simulink model "Project_HIL_Case_3"  (R2018b)
settings: Solver=ode5  StartTime=0.0  StopTime=180  FixedStep=0.01  RelTol=1e-3
InitFcn:
  | Initial_Data_Case_3
values from neighbouring files (symbols this model uses):
  alpha1 = 0.5    [Initial_Data_Case_3.m]
  alpha2 = 0.5    [Initial_Data_Case_3.m]
  alpha3 = 0.5    [Initial_Data_Case_3.m]
  gammadot_t = 0*pi/180    (= 0)    [Initial_Data_Case_3.m]
  landa1 = 1    [Initial_Data_Case_3.m]
  landa2 = 1    [Initial_Data_Case_3.m]
  landa3 = 1    [Initial_Data_Case_3.m]
  Vg_t = 10    [Initial_Data_Case_3.m]
undefined symbols (not defined in the file or in its folder): Serial_Port, Standard_Devices
libraries: svdutilitieslib x2, sldrtlib x2
settings Model: Creator=AmiR_KhaN  LastModifiedBy=AmiR_KhaN
settings DataIOCC: ReturnWorkspaceOutputs=on
settings RTWCC: Description=Simulink Desktop Real-Time  SystemTargetFile=sldrt.tlc  TemplateMakefile=sldrt.tmf  RTWCompilerOptimization=on
settings CodeAppCC: MaxIdLength=95
settings SimulinkDesktopRealTimeCC: TargetPreCompLibLocation=E:\programmes\newmatlab\toolbox\sldrt\lib\win64

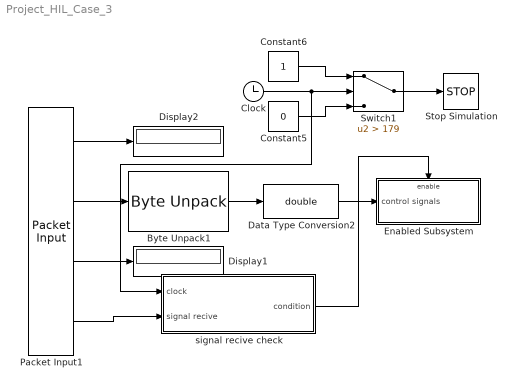
== system Project_HIL_Case_3 ==
  Byte Unpack1 : svdutilitieslib/Byte Unpack  dimensions={[3]}  datatypes={'single'}  byteAlign=1  blockPlatform=arduinoert
      settings: SourceProductBaseCode=ARDUINO,ML_ARDUINO,ECCORTEXA,ECCORTEXR,SC_BEAGLEBONE_BLUE,EC_FREEDOM_BOARD,EC_FRDM_K64F,INTEL_BLOCKSET,MICROBIT,NUCLEO,PX4AUTOPILOTS,RASPPIIO,STMICRODIS,TIC2000,XILINX_BLOCKSET
  Clock : Clock
  Constant5 : Constant  Value=0
  Constant6 : Constant
  Data Type Conversion2 : DataTypeConversion  OutDataTypeStr=double
  Display1 : Display
  Display2 : Display
  Enabled Subsystem : Subsystem  TreatAsAtomicUnit=on
  Packet Input1 : sldrtlib/Packet Input  SampleTime=0.01  MaxMissedTicks=10  ShowMissedTicks=off  YieldWhenWaiting=off  DrvName=Standard_Devices/Serial_Port  DrvAddress=5  DrvOptions=[9600 8 0 0 0 0 0 0]  PacketSize=14  DataTypes={'1*uint8','12*uint8','1*uint8'}  ShowReady=on  ShowError=off  PacketID=1  ByteOrder=1  ShowTimestamp=off
      settings: AttributesFormatString=Serial Port [5]
  Stop Simulation : Stop
  Switch1 : Switch  Criteria=u2 > Threshold  Threshold=179
  signal recive check : Subsystem
  wires:
  Packet Input1/1 -> Display2/1
  Packet Input1/3 -> Display1/1
  Clock/1 -> signal recive check/1(clock), Switch1/2
  Constant5/1 -> Switch1/3
  Data Type Conversion2/1 -> Enabled Subsystem/1(control signals)
  Constant6/1 -> Switch1/1
  Byte Unpack1/1 -> Data Type Conversion2/1
  Switch1/1 -> Stop Simulation/1
  Packet Input1/2 -> Byte Unpack1/1
  Packet Input1/4 -> signal recive check/2(signal recive)
  signal recive check/1(condition) -> Enabled Subsystem/Enable

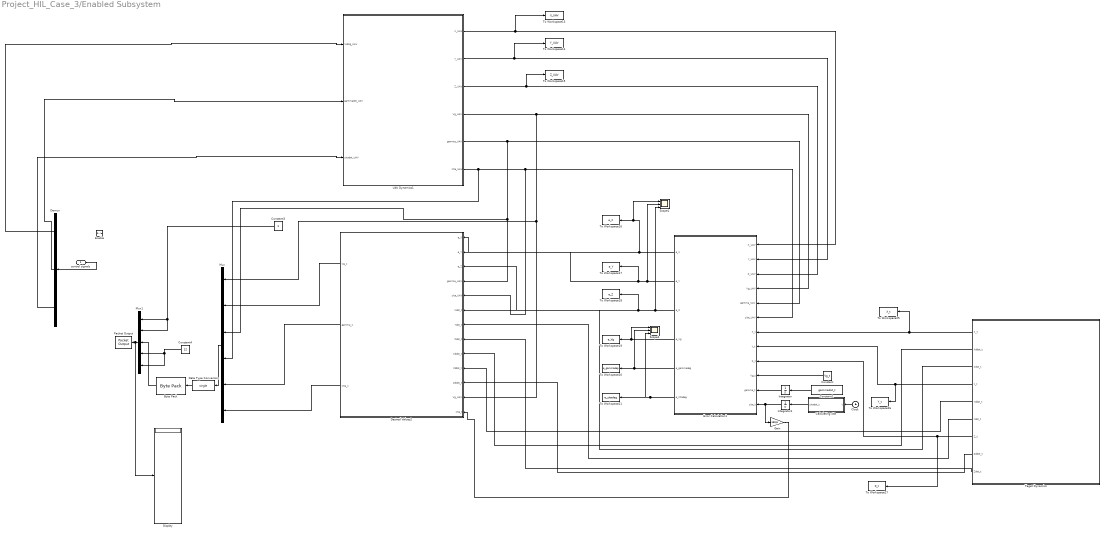
== system Project_HIL_Case_3/Enabled Subsystem ==
  control signals : Inport
  Enable : EnablePort
  Byte Pack : svdutilitieslib/Byte Pack  maskPackedDataType=uint8  datatypes={'single'}  byteAlign=4  blockPlatform=arduinoert
      settings: SourceProductBaseCode=ARDUINO,ML_ARDUINO,ECCORTEXA,ECCORTEXR,SC_BEAGLEBONE_BLUE,EC_FREEDOM_BOARD,EC_FRDM_K64F,INTEL_BLOCKSET,MICROBIT,NUCLEO,PX4AUTOPILOTS,RASPPIIO,STMICRODIS,TIC2000,XILINX_BLOCKSET
  Calculating zita : MATLAB Function  TreatAsAtomicUnit=on
  Clock : Clock
  Constant : Constant  Value=Vg_t
  Constant1 : Constant  Value=gammadot_t
  Constant3 : Constant  OutDataTypeStr=uint8
  Constant4 : Constant  Value=12  OutDataTypeStr=uint8
  Data Type Conversion : DataTypeConversion  OutDataTypeStr=single
  Demux : Demux  Outputs=3
  Desired Values2 : Subsystem
  Display : Display
  Error Calculation1 : MATLAB Function  TreatAsAtomicUnit=on
  Gain : Gain  Gain=180/pi
  Integrator : Integrator  InitialCondition=45*pi/180
  Integrator1 : Integrator  InitialCondition=0*pi/180
  Mux : Mux  Inputs=6
  Mux1 : Mux  Inputs=5
  Packet Output : sldrtlib/Packet Output  SampleTime=0.01  MaxMissedTicks=10  ShowMissedTicks=off  YieldWhenWaiting=off  DrvName=Standard_Devices/Serial_Port  DrvAddress=5  DrvOptions=[9600 8 0 0 0 0 0 0]  PacketSize=28  DataTypes='28*uint8'  ShowReady=off  ShowError=off  PacketID=1  ByteOrder=1  InitialValue=[]  FinalValue=[]
      settings: AttributesFormatString=Serial Port [5]
  Scope1 : Scope  NumInputPorts=3
  Scope2 : Scope  NumInputPorts=3
  Taget Dynamics : Subsystem
  To Workspace13 : ToWorkspace  VariableName=X_UAV  SaveFormat=Timeseries  SampleTime=-1
  To Workspace14 : ToWorkspace  VariableName=Y_UAV  SaveFormat=Timeseries  SampleTime=-1
  To Workspace15 : ToWorkspace  VariableName=Z_UAV  SaveFormat=Timeseries  SampleTime=-1
  To Workspace16 : ToWorkspace  VariableName=e_X  SaveFormat=Timeseries  SampleTime=-1
  To Workspace17 : ToWorkspace  VariableName=e_Y  SaveFormat=Timeseries  SampleTime=-1
  To Workspace18 : ToWorkspace  VariableName=e_Z  SaveFormat=Timeseries  SampleTime=-1
  To Workspace19 : ToWorkspace  VariableName=e_Vg  SaveFormat=Timeseries  SampleTime=-1
  To Workspace20 : ToWorkspace  VariableName=e_gammadeg  SaveFormat=Timeseries  SampleTime=-1
  To Workspace21 : ToWorkspace  VariableName=e_zitadeg  SaveFormat=Timeseries  SampleTime=-1
  To Workspace25 : ToWorkspace  VariableName=X_t  SaveFormat=Timeseries  SampleTime=-1
  To Workspace26 : ToWorkspace  VariableName=Y_t  SaveFormat=Timeseries  SampleTime=-1
  To Workspace27 : ToWorkspace  VariableName=Z_t  SaveFormat=Timeseries  SampleTime=-1
  UAV Dynamics1 : Subsystem
  wires:
  Desired Values2/3(zita_c) -> Mux/6
  control signals/1 -> Demux/1
  Constant4/1 -> Mux1/5, Mux1/4
  Demux/2 -> UAV Dynamics1/2(gammadot_UAV)
  Demux/1 -> UAV Dynamics1/1(Vdotg_UAV)
  Demux/3 -> UAV Dynamics1/3(zitadot_UAV)
  Data Type Conversion/1 -> Byte Pack/1
  Mux1/1 -> Display/1, Packet Output/1
  Mux/1 -> Data Type Conversion/1
  Byte Pack/1 -> Mux1/3
  Desired Values2/1(Vg_c) -> Mux/2
  Desired Values2/2(gamma_c) -> Mux/5
  UAV Dynamics1/6(zita_UAV) -> Mux/4, Desired Values2/5(zita_UAV), Error Calculation1/6(zita_UAV)
  Taget Dynamics/7(Z_t) -> To Workspace27/1, Error Calculation1/9(Z_t)
  Taget Dynamics/1(X_t) -> To Workspace25/1, Error Calculation1/7(X_t)
  Taget Dynamics/5(Yddot_t) -> Desired Values2/10(Yddot_t)
  Taget Dynamics/2(Xddot_t) -> Desired Values2/9(Xddot_t)
  Constant/1 -> Error Calculation1/10(Vg_t)
  Clock/1 -> Calculating zita/1(t)
  Taget Dynamics/6(Ydot_t) -> Desired Values2/7(Ydot_t)
  Taget Dynamics/4(Y_t) -> To Workspace26/1, Error Calculation1/8(Y_t)
  Taget Dynamics/9(Zdot_t) -> Desired Values2/8(Zdot_t)
  Taget Dynamics/3(Xdot_t) -> Desired Values2/6(Xdot_t)
  UAV Dynamics1/3(Z_UAV) -> To Workspace15/1, Error Calculation1/3(Z_UAV)
  Constant1/1 -> Integrator/1
  Taget Dynamics/8(Zddot_t) -> Desired Values2/11(Zddot_t)
  Calculating zita/1(zitadot_t) -> Integrator1/1
  UAV Dynamics1/2(Y_UAV) -> To Workspace14/1, Error Calculation1/2(Y_UAV)
  Gain/1 -> Desired Values2/13(zita_t)
  UAV Dynamics1/1(X_UAV) -> To Workspace13/1, Error Calculation1/1(X_UAV)
  Integrator1/1 -> Error Calculation1/12(zita_t), Gain/1
  UAV Dynamics1/5(gamma_UAV) -> Mux/3, Desired Values2/4(gamma_UAV), Error Calculation1/5(gamma_UAV)
  Integrator/1 -> Error Calculation1/11(gamma_t)
  UAV Dynamics1/4(Vg_UAV) -> Mux/1, Desired Values2/12(Vg_UAV), Error Calculation1/4(Vg_UAV)
  Constant3/1 -> Mux1/2, Mux1/1
  Error Calculation1/4(e_Vg) -> Scope2/1, To Workspace19/1
  Error Calculation1/6(e_zitadeg) -> Scope2/3, To Workspace21/1
  Error Calculation1/5(e_gammadeg) -> Scope2/2, To Workspace20/1
  Error Calculation1/1(e_X) -> Desired Values2/1(e_X), Scope1/1, To Workspace16/1
  Error Calculation1/3(e_Z) -> Scope1/3, Desired Values2/3(e_Z), To Workspace18/1
  Error Calculation1/2(e_Y) -> Scope1/2, Desired Values2/2(e_Y), To Workspace17/1

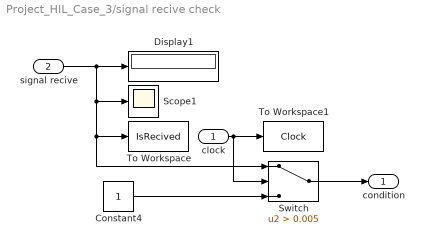
== system Project_HIL_Case_3/signal recive check ==
  clock : Inport
  signal recive : Inport  Port=2
  Constant4 : Constant
  Display1 : Display
  Scope1 : Scope
  Switch : Switch  Criteria=u2 > Threshold  Threshold=0.005
  To Workspace : ToWorkspace  VariableName=IsRecived  SampleTime=-1
  To Workspace1 : ToWorkspace  VariableName=Clock  SampleTime=-1
  condition : Outport
  wires:
  signal recive/1 -> Switch/1, To Workspace/1, Scope1/1, Display1/1
  Switch/1 -> condition/1
  clock/1 -> Switch/2, To Workspace1/1
  Constant4/1 -> Switch/3

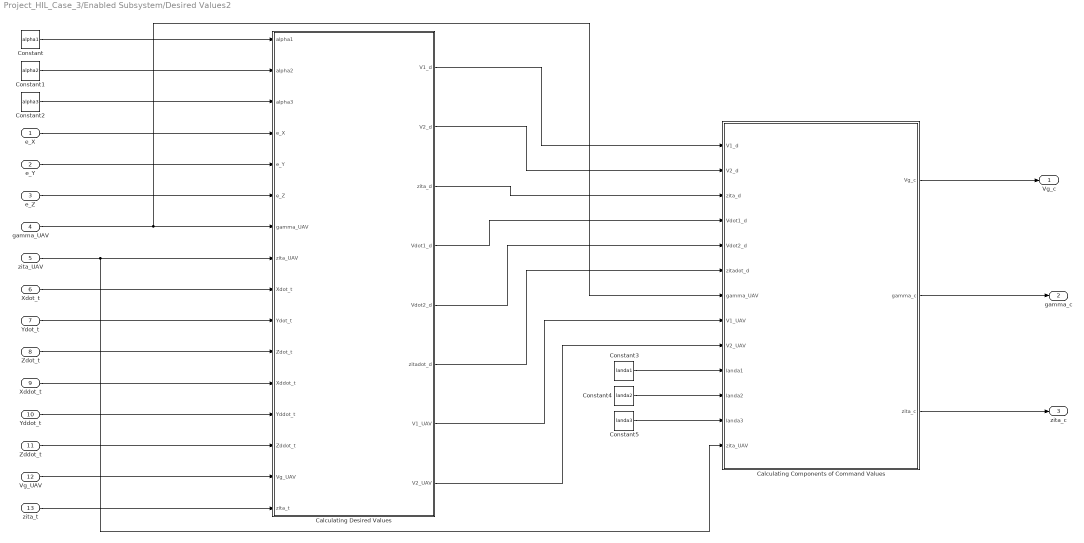
== system Project_HIL_Case_3/Enabled Subsystem/Desired Values2 ==
  e_X : Inport
  e_Y : Inport  Port=2
  e_Z : Inport  Port=3
  gamma_UAV : Inport  Port=4
  zita_UAV : Inport  Port=5
  Xdot_t : Inport  Port=6
  Ydot_t : Inport  Port=7
  Zdot_t : Inport  Port=8
  Xddot_t : Inport  Port=9
  Yddot_t : Inport  Port=10
  Zddot_t : Inport  Port=11
  Vg_UAV : Inport  Port=12
  zita_t : Inport  Port=13
  Calculating Components of Command Values : MATLAB Function  TreatAsAtomicUnit=on
  Calculating Desired Values : MATLAB Function  TreatAsAtomicUnit=on
  Constant : Constant  Value=alpha1
  Constant1 : Constant  Value=alpha2
  Constant2 : Constant  Value=alpha3
  Constant3 : Constant  Value=landa1
  Constant4 : Constant  Value=landa2
  Constant5 : Constant  Value=landa3
  Vg_c : Outport  VectorParamsAs1DForOutWhenUnconnected=off
  gamma_c : Outport  Port=2  VectorParamsAs1DForOutWhenUnconnected=off
  zita_c : Outport  Port=3  VectorParamsAs1DForOutWhenUnconnected=off
  wires:
  Constant/1 -> Calculating Desired Values/1(alpha1)
  Constant1/1 -> Calculating Desired Values/2(alpha2)
  Constant2/1 -> Calculating Desired Values/3(alpha3)
  e_X/1 -> Calculating Desired Values/4(e_X)
  e_Y/1 -> Calculating Desired Values/5(e_Y)
  e_Z/1 -> Calculating Desired Values/6(e_Z)
  gamma_UAV/1 -> Calculating Desired Values/7(gamma_UAV), Calculating Components of Command Values/7(gamma_UAV)
  zita_UAV/1 -> Calculating Desired Values/8(zita_UAV), Calculating Components of Command Values/13(zita_UAV)
  Xdot_t/1 -> Calculating Desired Values/9(Xdot_t)
  Ydot_t/1 -> Calculating Desired Values/10(Ydot_t)
  Zdot_t/1 -> Calculating Desired Values/11(Zdot_t)
  Xddot_t/1 -> Calculating Desired Values/12(Xddot_t)
  Yddot_t/1 -> Calculating Desired Values/13(Yddot_t)
  Zddot_t/1 -> Calculating Desired Values/14(Zddot_t)
  Vg_UAV/1 -> Calculating Desired Values/15(Vg_UAV)
  Calculating Desired Values/1(V1_d) -> Calculating Components of Command Values/1(V1_d)
  Calculating Desired Values/2(V2_d) -> Calculating Components of Command Values/2(V2_d)
  Calculating Desired Values/3(zita_d) -> Calculating Components of Command Values/3(zita_d)
  Calculating Desired Values/4(Vdot1_d) -> Calculating Components of Command Values/4(Vdot1_d)
  Calculating Desired Values/5(Vdot2_d) -> Calculating Components of Command Values/5(Vdot2_d)
  Calculating Desired Values/6(zitadot_d) -> Calculating Components of Command Values/6(zitadot_d)
  Calculating Desired Values/7(V1_UAV) -> Calculating Components of Command Values/8(V1_UAV)
  Calculating Desired Values/8(V2_UAV) -> Calculating Components of Command Values/9(V2_UAV)
  Constant3/1 -> Calculating Components of Command Values/10(landa1)
  Constant4/1 -> Calculating Components of Command Values/11(landa2)
  Constant5/1 -> Calculating Components of Command Values/12(landa3)
  Calculating Components of Command Values/1(Vg_c) -> Vg_c/1
  Calculating Components of Command Values/2(gamma_c) -> gamma_c/1
  Calculating Components of Command Values/3(zita_c) -> zita_c/1
  zita_t/1 -> Calculating Desired Values/16(zita_t)

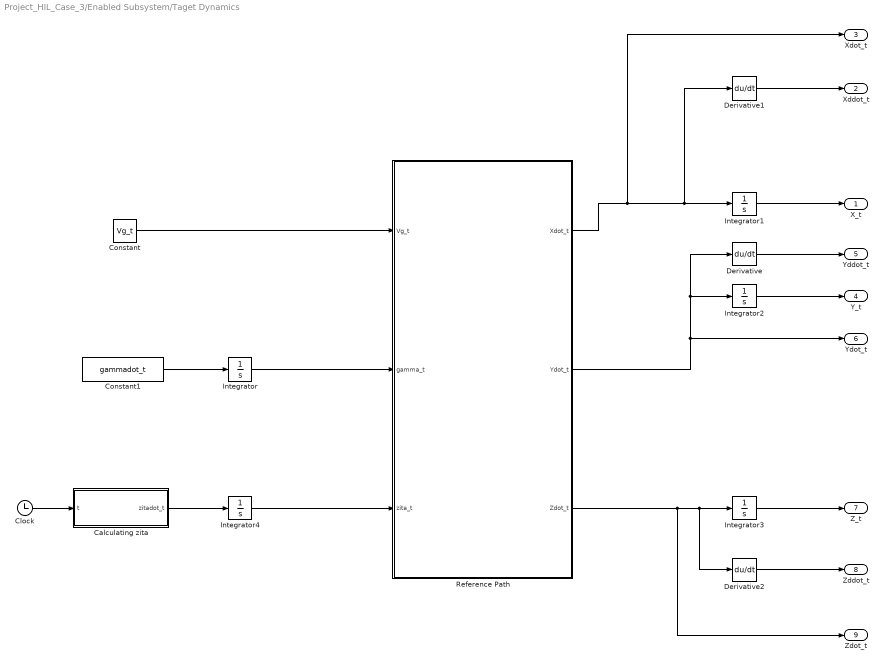
== system Project_HIL_Case_3/Enabled Subsystem/Taget Dynamics ==
  Calculating zita : MATLAB Function  TreatAsAtomicUnit=on
  Clock : Clock
  Constant : Constant  Value=Vg_t
  Constant1 : Constant  Value=gammadot_t
  Derivative : Derivative
  Derivative1 : Derivative
  Derivative2 : Derivative
  Integrator : Integrator  InitialCondition=45*pi/180
  Integrator1 : Integrator  InitialCondition=100
  Integrator2 : Integrator  InitialCondition=100
  Integrator3 : Integrator  InitialCondition=100
  Integrator4 : Integrator  InitialCondition=0*pi/180
  Reference Path : MATLAB Function  TreatAsAtomicUnit=on
  X_t : Outport  VectorParamsAs1DForOutWhenUnconnected=off
  Xddot_t : Outport  Port=2  VectorParamsAs1DForOutWhenUnconnected=off
  Xdot_t : Outport  Port=3  VectorParamsAs1DForOutWhenUnconnected=off
  Y_t : Outport  Port=4  VectorParamsAs1DForOutWhenUnconnected=off
  Yddot_t : Outport  Port=5  VectorParamsAs1DForOutWhenUnconnected=off
  Ydot_t : Outport  Port=6  VectorParamsAs1DForOutWhenUnconnected=off
  Z_t : Outport  Port=7  VectorParamsAs1DForOutWhenUnconnected=off
  Zddot_t : Outport  Port=8  VectorParamsAs1DForOutWhenUnconnected=off
  Zdot_t : Outport  Port=9  VectorParamsAs1DForOutWhenUnconnected=off
  wires:
  Integrator1/1 -> X_t/1
  Derivative1/1 -> Xddot_t/1
  Reference Path/1(Xdot_t) -> Derivative1/1, Integrator1/1, Xdot_t/1
  Integrator2/1 -> Y_t/1
  Reference Path/2(Ydot_t) -> Integrator2/1, Derivative/1, Ydot_t/1
  Derivative/1 -> Yddot_t/1
  Reference Path/3(Zdot_t) -> Zdot_t/1, Derivative2/1, Integrator3/1
  Derivative2/1 -> Zddot_t/1
  Integrator3/1 -> Z_t/1
  Integrator/1 -> Reference Path/2(gamma_t)
  Constant/1 -> Reference Path/1(Vg_t)
  Constant1/1 -> Integrator/1
  Clock/1 -> Calculating zita/1(t)
  Calculating zita/1(zitadot_t) -> Integrator4/1
  Integrator4/1 -> Reference Path/3(zita_t)

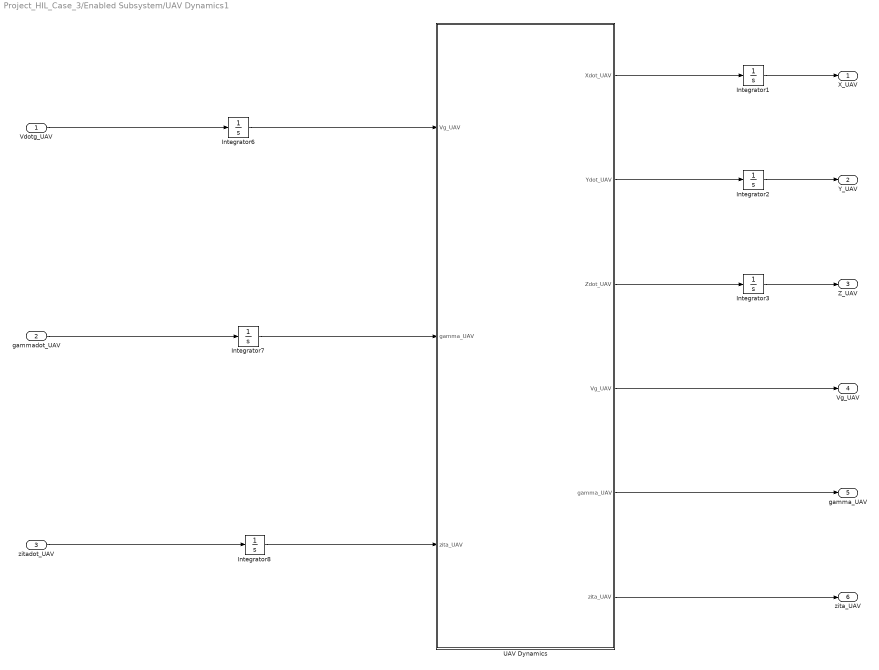
== system Project_HIL_Case_3/Enabled Subsystem/UAV Dynamics1 ==
  Vdotg_UAV : Inport
  gammadot_UAV : Inport  Port=2
  zitadot_UAV : Inport  Port=3
  Integrator1 : Integrator  InitialCondition=80
  Integrator2 : Integrator  InitialCondition=90
  Integrator3 : Integrator  InitialCondition=70
  Integrator6 : Integrator  InitialCondition=8
  Integrator7 : Integrator  InitialCondition=0*pi/180
  Integrator8 : Integrator  InitialCondition=0*pi/180
  UAV Dynamics : MATLAB Function  TreatAsAtomicUnit=on
  X_UAV : Outport  VectorParamsAs1DForOutWhenUnconnected=off
  Y_UAV : Outport  Port=2  VectorParamsAs1DForOutWhenUnconnected=off
  Z_UAV : Outport  Port=3  VectorParamsAs1DForOutWhenUnconnected=off
  Vg_UAV : Outport  Port=4  VectorParamsAs1DForOutWhenUnconnected=off
  gamma_UAV : Outport  Port=5  VectorParamsAs1DForOutWhenUnconnected=off
  zita_UAV : Outport  Port=6  VectorParamsAs1DForOutWhenUnconnected=off
  wires:
  Integrator3/1 -> Z_UAV/1
  UAV Dynamics/1(Xdot_UAV) -> Integrator1/1
  Integrator2/1 -> Y_UAV/1
  UAV Dynamics/2(Ydot_UAV) -> Integrator2/1
  UAV Dynamics/3(Zdot_UAV) -> Integrator3/1
  Integrator1/1 -> X_UAV/1
  UAV Dynamics/4(Vg_UAV) -> Vg_UAV/1
  UAV Dynamics/5(gamma_UAV) -> gamma_UAV/1
  UAV Dynamics/6(zita_UAV) -> zita_UAV/1
  Vdotg_UAV/1 -> Integrator6/1
  Integrator6/1 -> UAV Dynamics/1("Vg_UAV ")
  gammadot_UAV/1 -> Integrator7/1
  Integrator7/1 -> UAV Dynamics/2("gamma_UAV ")
  zitadot_UAV/1 -> Integrator8/1
  Integrator8/1 -> UAV Dynamics/3("zita_UAV ")

== matlab function Project_HIL_Case_3/Enabled Subsystem/Taget Dynamics/Calculating zita ==
  data: t input; zitadot_t output
function zitadot_t = fcn(t)

zitadot_t = sin((2*pi/30)*t);

== matlab function Project_HIL_Case_3/Enabled Subsystem/Calculating zita ==
  data: t input; zitadot_t output
function zitadot_t = fcn(t)

zitadot_t = sin((2*pi/30)*t);

== matlab function Project_HIL_Case_3/Enabled Subsystem/Desired Values2/Calculating Components of Command Values ==
  data: V1_d input; Vg_c output; V2_d input; zita_d input; Vdot1_d input; Vdot2_d input; zitadot_d input; gamma_UAV input; V1_UAV input; V2_UAV input; landa1 input; landa2 input; landa3 input; gamma_c output; zita_c output; zita_UAV input
function [Vg_c,gamma_c,zita_c] = fcn(V1_d,V2_d,zita_d,Vdot1_d,Vdot2_d,zitadot_d,gamma_UAV, V1_UAV,V2_UAV,landa1,landa2,landa3,zita_UAV)

Vg_c1 = -Vdot1_d + landa1*(V1_UAV - V1_d);
Vg_c2 = -Vdot2_d + landa2*(V2_UAV - V2_d);
Vg_c = Vg_c1*cos(gamma_UAV) + Vg_c2*sin(gamma_UAV);
gamma_c1 = -Vdot1_d + landa1*(V1_UAV - V1_d);
gamma_c2 = -Vdot2_d + landa2*(V2_UAV - V2_d);
gamma_c = -sin(gamma_UAV)*gamma_c1 + cos(gamma_UAV)*gamma_c2;
zita_c = -zitadot_d + landa3*(zita_UAV - zita_d);

== matlab function Project_HIL_Case_3/Enabled Subsystem/Desired Values2/Calculating Desired Values ==
  data: alpha1 input; V1_d output; V2_d output; zita_d output; Vdot1_d output; Vdot2_d output; zitadot_d output; alpha2 input; alpha3 input; e_X input; e_Y input; e_Z input; gamma_UAV input; zita_UAV input; Xdot_t input; Ydot_t input; Zdot_t input; Xddot_t input; Yddot_t input; Zddot_t input; Vg_UAV input; V1_UAV output; V2_UAV output; zita_t input
function [V1_d,V2_d,zita_d,Vdot1_d,Vdot2_d,zitadot_d,V1_UAV,V2_UAV] = fcn(alpha1,alpha2,alpha3,e_X,e_Y,e_Z,gamma_UAV,zita_UAV,Xdot_t,Ydot_t,Zdot_t,Xddot_t,Yddot_t,Zddot_t,Vg_UAV,zita_t)

V1_UAV = Vg_UAV*cos(gamma_UAV);
V2_UAV = Vg_UAV*sin(gamma_UAV);
V1_d = sqrt((-alpha1*e_X + Xdot_t)^2 + (-alpha2*e_Y + Ydot_t)^2);
V2_d = -alpha3*e_Z + Zdot_t;
y = (-alpha2*e_Y + Ydot_t);
x = (-alpha1*e_X + Xdot_t);
zita_d = atan2(y,x);

% T = 15; % Period the time that takes for zita_t to reach 180 degree
% 
if y < 0 && zita_t >= 180
     zita_d = 2*pi + zita_d;
 end

if y > 0 && zita_t >= 360
    zita_d = 2*pi + zita_d;
end

if y < 0 && zita_t >= 540
    zita_d = 2*pi + zita_d;
end

Vdot1_d = (1/V1_d)*((-alpha1*e_X + Xdot_t)*(-alpha1*V1_UAV*cos(zita_UAV) + Xddot_t + alpha1*Xdot_t) + (-alpha2*e_Y + Ydot_t)*(-alpha2*V1_UAV*sin(zita_UAV) + Yddot_t + alpha2*Ydot_t));
Vdot2_d = -alpha3*V2_UAV + Zddot_t + alpha3*Zdot_t;
zitadot_d = (1/V1_d)*(cos(zita_d)*(-alpha2*V1_UAV*sin(zita_UAV) + Yddot_t + alpha2*Ydot_t) - sin(zita_d)*(-alpha1*V1_UAV*cos(zita_UAV) + Xddot_t + alpha1*Xdot_t));

== matlab function Project_HIL_Case_3/Enabled Subsystem/Error Calculation1 ==
  data: X_UAV input; e_X output; Y_UAV input; Z_UAV input; Vg_UAV input; gamma_UAV input; zita_UAV input; X_t input; Y_t input; Z_t input; Vg_t input; gamma_t input; zita_t input; e_Y output; e_Z output; e_Vg output; e_gammadeg output; e_zitadeg output
function [e_X,e_Y,e_Z,e_Vg,e_gammadeg,e_zitadeg] = fcn(X_UAV,Y_UAV,Z_UAV,Vg_UAV,gamma_UAV,zita_UAV,X_t,Y_t,Z_t,Vg_t,gamma_t,zita_t)

e_X = X_UAV - X_t;
e_Y = Y_UAV - Y_t;
e_Z = Z_UAV - Z_t;
e_Vg = Vg_UAV - Vg_t;
e_gamma = gamma_UAV - gamma_t;
e_zita = zita_UAV - zita_t;
e_gammadeg = e_gamma*(180/pi);
e_zitadeg = e_zita*(180/pi);

== matlab function Project_HIL_Case_3/Enabled Subsystem/Taget Dynamics/Reference Path ==
  data: Vg_t input; Xdot_t output; gamma_t input; zita_t input; Ydot_t output; Zdot_t output
function [Xdot_t,Ydot_t,Zdot_t]  = fcn(Vg_t,gamma_t,zita_t)

Xdot_t = Vg_t*cos(gamma_t)*cos(zita_t);
Ydot_t = Vg_t*cos(gamma_t)*sin(zita_t);
Zdot_t = Vg_t*sin(gamma_t);

== matlab function Project_HIL_Case_3/Enabled Subsystem/UAV Dynamics1/UAV Dynamics ==
  data: Xdot_UAV output; Ydot_UAV output; Vg_UAV input; Zdot_UAV output; gamma_UAV input; zita_UAV input; Vg_UAV output; gamma_UAV output; zita_UAV output
function [Xdot_UAV,Ydot_UAV,Zdot_UAV,Vg_UAV,gamma_UAV,zita_UAV]  = fcn(Vg_UAV,gamma_UAV,zita_UAV)

Xdot_UAV = Vg_UAV*cos(gamma_UAV)*cos(zita_UAV);
Ydot_UAV = Vg_UAV*cos(gamma_UAV)*sin(zita_UAV);
Zdot_UAV = Vg_UAV*sin(gamma_UAV);
